simulink model "untitled_yuv"  (R2021a)
settings: Solver=VariableStepAuto  StartTime=0.0  StopTime=10.0  RelTol=1e-3
libraries: mpcadaslib x1
settings Model: Creator=yuval  LastModifiedBy=yuval

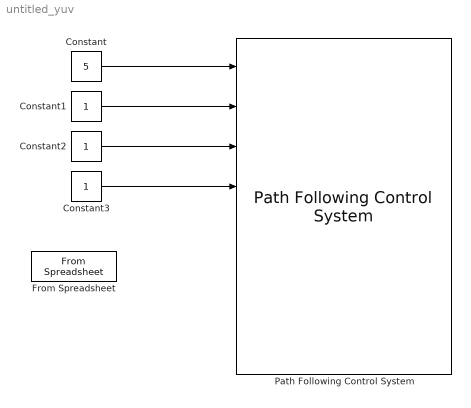
== system untitled_yuv ==
  Constant : Constant  Value=5
  Constant1 : Constant
  Constant2 : Constant
  Constant3 : Constant
  From Spreadsheet : FromSpreadsheet
  Path Following Control System : mpcadaslib/Path Following Control System  VariantControl=Variant2  ModelType=Use vehicle parameters  VehicleMass=1575  VehicleYawInertia=2875  LengthToFront=1.2  LengthToRear=1.6  FrontTireStiffness=19000  RearTireStiffness=33000  AccelTimeConstant=0.5  EgoModelMatrixA=[-2,zeros(1,3);1,zeros(1,3);zeros(1,2),-4.4021,-12.4603;zeros(1,2),1.3913,-5.1868]  EgoModelMatrixB=[2,zeros(1,3);zeros(1,2),24.1270,15.8609]'  EgoModelMatrixC=[zeros(3,1),eye(3)]  InitialLongVel=15  TransportLag=0  spaceCtrl=on  DefaultSpacing=10  MinSteering=-0.26  umin_ext=off  MaxSteering=0.26  umax_ext=off  MinAcceleration=-3  amin_ext=off  MaxAcceleration=2  amax_ext=off  Ts=0.05  PredictionHorizon=40  ControlHorizon=1  LongWeight=0.1  LateralWeight=1  AccelRateWeight=0.1  SteerRateWeight=0.1  suboptimal=off  maxiter=10  datatypeopt=double  optmode=off  trackmode=off
      settings: SourceProductBaseCode=MP
  wires:
  Constant/1 -> Path Following Control System/1
  Constant1/1 -> Path Following Control System/2
  Constant2/1 -> Path Following Control System/3
  Constant3/1 -> Path Following Control System/4
